simulink model "IM_RFOC_controller_sim"  (R2023a)
settings: Solver=ode23t  StartTime=0.0  StopTime=50  RelTol=1e-3
values from neighbouring files (symbols this model uses):
  B = 0.068    [IM_model_parameters.m]
  f = 50    [IM_model_parameters.m]
  isq_n = 1.278    [IM_model_parameters.m]
  J = 0.4    [IM_model_parameters.m]
  k = 0.009    [IM_model_parameters.m]
  kicdq = 41.5*100    (= 4150)    [IM_model_parameters.m]
  kiw = 0.068*1000    (= 68)    [IM_model_parameters.m]
  kiYr = 17.54286*1000    (= 17542.86)    [IM_model_parameters.m]
  kpcdq = .4425*100    (= 44.25)    [IM_model_parameters.m]
  kpw = 0.4*1000    (= 400)    [IM_model_parameters.m]
  kpYr = 5.71429*1000    (= 5714.29)    [IM_model_parameters.m]
  Lks = Ls- Lm^2/Lr    (= 0.00442538071066)    [IM_model_parameters.m]
  Lm = 57e-3    (= 0.057)    [IM_model_parameters.m]
  np = 3    [IM_model_parameters.m]
  r = 4    [IM_model_parameters.m]
  Rr = 0.175    [IM_model_parameters.m]
  Rs = 0.24    [IM_model_parameters.m]
  vsat = 380    [IM_model_parameters.m]
  Yrd_n = 1.9373    [IM_model_parameters.m]
undefined symbols (not defined in the file or in its folder): j, magnitude
libraries: slpidlib x4, eeTransforms x4, simulink x1
settings Model: Creator=Andrea  LastModifiedBy=Andrea
settings SolverCC: ZeroCrossAlgorithm=Adaptive
settings OptimizationCC: ReuseModelBlockBuffer=off

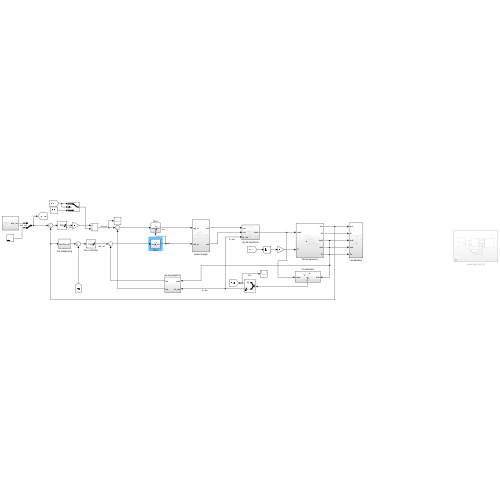
[thumbnail: Simulink's stored preview of the top-level diagram]
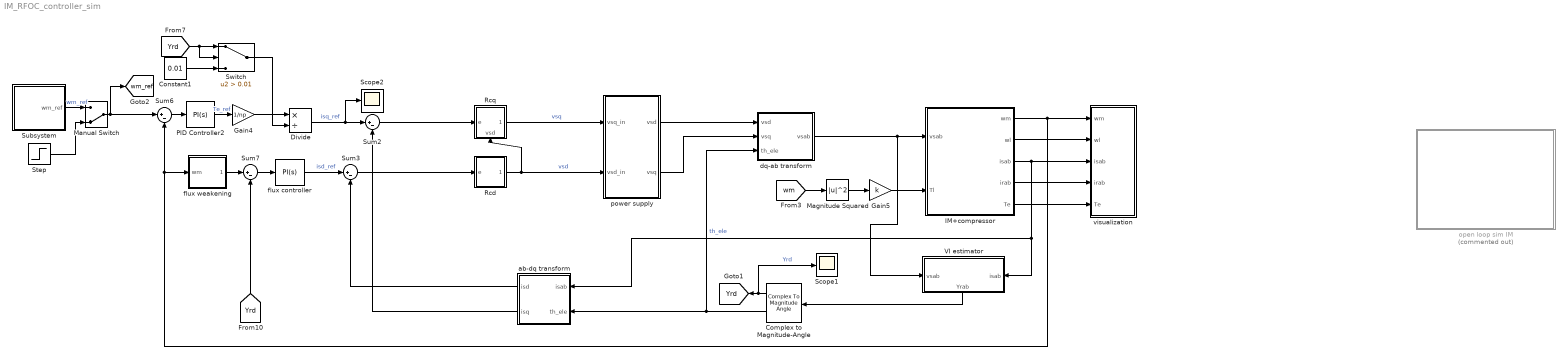
== system IM_RFOC_controller_sim ==
  Complex to Magnitude-Angle : ComplexToMagnitudeAngle
  Constant1 : Constant  Value=0.01
  Divide : Product  Inputs=*/  RndMeth=Zero  SaturateOnIntegerOverflow=on
  Gain4 : Gain  Gain=1/np
  Gain5 : Gain  Gain=k
  IM+compressor : Subsystem
  Magnitude Squared : Math  Operator=magnitude^2
  Manual Switch : ManualSwitch  CurrentSetting=0
  PID Controller2 : slpidlib/PID Controller  Controller=PI  Form=Parallel  TimeDomain=Continuous-time  UseExternalTs=off  SampleTime=-1  IntegratorMethod=Forward Euler  FilterMethod=Forward Euler  ControllerParametersSource=internal  P=kpw  I=kiw  UseKiTs=off  D=0  N=100  UseFilter=on  TunerSelectOption=Transfer Function Based (PID Tuner App)  InitialConditionSource=internal  InitialConditionForIntegrator=0  InitialConditionForFilter=0  DifferentiatorICPrevScaledInput=0  ExternalReset=none  TrackingMode=off  Kt=1  LimitOutput=on  SatLimitsSource=internal  UpperSaturationLimit=1000  LowerSaturationLimit=-1000  LinearizeAsGain=on  AntiWindupMode=back-calculation  Kb=kiw/kpw  LimitIntegrator=off  UpperIntegratorSaturationLimit=inf  LowerIntegratorSaturationLimit=-inf  POutMin=[]  POutMax=[]  IOutMin=[]  IOutMax=[]  DOutMin=[]  DOutMax=[]  NOutMin=[]  NOutMax=[]  SumOutMin=[]  SumOutMax=[]  SaturationOutMin=[]  SaturationOutMax=[]  PParamMin=[]  PParamMax=[]  IParamMin=[]  IParamMax=[]  DParamMin=[]  DParamMax=[]  NParamMin=[]  NParamMax=[]  KbParamMin=[]  KbParamMax=[]  KtParamMin=[]  KtParamMax=[]  KbOutMin=[]  KbOutMax=[]  KtOutMin=[]  KtOutMax=[]  IntegratorOutMin=[]  IntegratorOutMax=[]  FilterOutMin=[]  FilterOutMax=[]  SumI1OutMin=[]  SumI1OutMax=[]  SumI2OutMin=[]  SumI2OutMax=[]  SumI3OutMin=[]  SumI3OutMax=[]  SumI4OutMin=[]  SumI4OutMax=[]  SumDOutMin=[]  SumDOutMax=[]  DifferentiatorOutMin=[]  DifferentiatorOutMax=[]  FilterDiffOutCoefMin=[]  FilterDiffOutCoefMax=[]  ReciprocalOutMin=[]  ReciprocalOutMax=[]  SumDenOutMin=[]  SumDenOutMax=[]  SumNumOutMin=[]  SumNumOutMax=[]  DivideOutMin=[]  DivideOutMax=[]  UdiffTsProdOutMin=[]  UdiffTsProdOutMax=[]  NTsProdOutMin=[]  NTsProdOutMax=[]  UintegralTsProdOutMin=[]  UintegralTsProdOutMax=[]  UngainTsProdOutMin=[]  UngainTsProdOutMax=[]  ClampingZeroOutDataTypeStr=Inherit: Inherit via back propagation  ClampingZeroOutMin=[]  ClampingZeroOutMax=[]  FilterDenConstantOutDataTypeStr=Inherit: Inherit via back propagation  FilterDenConstantOutMin=[]  FilterDenConstantOutMax=[]  PCopyOutDataTypeStr=Inherit: Inherit via back propagation  PCopyOutMin=[]  PCopyOutMax=[]  NCopyOutDataTypeStr=Inherit: Inherit via back propagation  NCopyOutMin=[]  NCopyOutMax=[]  IntegratorContinuousStateAttributes=''  IntegratorStateMustResolveToSignalObject=off  IntegratorRTWStateStorageClass=Auto  FilterContinuousStateAttributes=''  FilterStateMustResolveToSignalObject=off  FilterRTWStateStorageClass=Auto  ParallelPVariant=InternalParameters  IdealPVariant=Disabled  IVariant=InternalParameters  DVariant=Disabled  IntegratorVariant=Continuous  SatVariant=Enabled  AWVariant=BackCalculation  PCopyVariant=Disabled  TRVariant=Disabled  FdbkBlocksVariant=Forward  IdealPFdbkVariant=Disabled  SatFdbkVariant=Disabled  DerivativeFilterVariant=Disabled  NVariant=Disabled  NCopyVariant=Disabled_SignalSpec  FilterICVariant=Disabled  IntegratorICVariant=InternalICs  ExternalResetVariant=Disabled  TRSumVariant=Passthrough  SumFdbkVariant=Disabled  SumVariant=Sum_PI  TsampFilterVariant=InternalTs  TsampNgainVariant=Passthrough  TsampIntegralVariant=Disabled_SignalSpec  ExternalSaturationOutDataTypeStr=Inherit: Same as second input
  Rcd : Subsystem
  Rcq : Subsystem
      settings: PortSchema="{\"entries\":[{\"content\":{\"sides\":[{\"content\":{\"connectorIds\":[\"In1\"]},\"type\":\"ConnectorPlacement.EquallySpacedRectSide\",\"uuid\":\"4a0c1cc3-c5ad-4afb-85ab-da55195444c6\"},{\"content\":{\"connectorIds\":[\"Out1\"],\"side\":\"RIGHT\"},\"type\":\"ConnectorPlacement.EquallySpacedRectSide\",\"uuid\":\"d24be668-1d0c-4d32-ba8c-18ff6b5ffdfe\"},{\"content\":{\"side\":\"TOP\"},\"type\":\"ConnectorPlacement.EquallySpacedRectSide\",\"uuid\":\"149b91f5-2af2-4df5-b968-7fe381dfd022\"},{\"content\":{\"connectorIds\":[\"In2\"],\"side\":\"BOTTOM\"},\"type\":\"ConnectorPlacement.EquallySpacedRectSide\",\"uuid\":\"c725719b-4b0c-406e-92d6-5caa670663a4\"}]},\"type\":\"ConnectorPlacement.EquallySpacedConnector\",\"uuid\":\"0f41f2af-cb74-4ff9-b902-e7fe768cb33d\"}],\"packageUris\":[\"http://schema.mathworks.com/mf0/Connector/R2020b\"],\"version\":\"1.0\"}"
  Scope1 : Scope
  Scope2 : Scope
  Step : Step  Time=2  After=200  SampleTime=0
  Subsystem : Subsystem
  Sum{2..3,6..7} (4 alike) : Sum  Inputs=|+-
  Switch : Switch  Criteria=u2 > Threshold  Threshold=0.01  SaturateOnIntegerOverflow=off  InputSameDT=off
  VI estimator : Subsystem
      settings: PortSchema="{\"entries\":[{\"content\":{\"sides\":[{\"content\":{},\"type\":\"ConnectorPlacement.EquallySpacedRectSide\",\"uuid\":\"e33eea5d-c803-4efd-b963-b28e7fd3b846\"},{\"content\":{\"connectorIds\":[\"Out1\"],\"side\":\"RIGHT\"},\"type\":\"ConnectorPlacement.EquallySpacedRectSide\",\"uuid\":\"16dd9f0c-f93f-4294-bb00-4f02950fe655\"},{\"content\":{\"connectorIds\":[\"In1\"],\"side\":\"TOP\"},\"type\":\"ConnectorPlacement.EquallySpacedRectSide\",\"uuid\":\"0c6e3d24-7610-41dc-8be5-eb5e396d3954\"},{\"content\":{\"connectorIds\":[\"In2\"],\"side\":\"BOTTOM\"},\"type\":\"ConnectorPlacement.EquallySpacedRectSide\",\"uuid\":\"785fd01a-f2d8-4593-9bc3-fce65e17d3d8\"}]},\"type\":\"ConnectorPlacement.EquallySpacedConnector\",\"uuid\":\"dc648cf4-6df6-4217-8a75-6fc5bc573b99\"}],\"packageUris\":[\"http://schema.mathworks.com/mf0/Connector/R2020b\"],\"version\":\"1.0\"}"
  ab-dq transform : Subsystem
  dq-ab transform : Subsystem
  flux controller : slpidlib/PID Controller  Controller=PI  Form=Parallel  TimeDomain=Continuous-time  UseExternalTs=off  SampleTime=-1  IntegratorMethod=Forward Euler  FilterMethod=Forward Euler  ControllerParametersSource=internal  P=kpYr  I=kiYr  UseKiTs=off  D=0  N=100  UseFilter=on  TunerSelectOption=Transfer Function Based (PID Tuner App)  InitialConditionSource=internal  InitialConditionForIntegrator=0  InitialConditionForFilter=0  DifferentiatorICPrevScaledInput=0  ExternalReset=none  TrackingMode=off  Kt=1  LimitOutput=on  SatLimitsSource=internal  UpperSaturationLimit=50  LowerSaturationLimit=-50  LinearizeAsGain=on  AntiWindupMode=back-calculation  Kb=kiYr/kpYr  LimitIntegrator=off  UpperIntegratorSaturationLimit=inf  LowerIntegratorSaturationLimit=-inf  POutMin=[]  POutMax=[]  IOutMin=[]  IOutMax=[]  DOutMin=[]  DOutMax=[]  NOutMin=[]  NOutMax=[]  SumOutMin=[]  SumOutMax=[]  SaturationOutMin=[]  SaturationOutMax=[]  PParamMin=[]  PParamMax=[]  IParamMin=[]  IParamMax=[]  DParamMin=[]  DParamMax=[]  NParamMin=[]  NParamMax=[]  KbParamMin=[]  KbParamMax=[]  KtParamMin=[]  KtParamMax=[]  KbOutMin=[]  KbOutMax=[]  KtOutMin=[]  KtOutMax=[]  IntegratorOutMin=[]  IntegratorOutMax=[]  FilterOutMin=[]  FilterOutMax=[]  SumI1OutMin=[]  SumI1OutMax=[]  SumI2OutMin=[]  SumI2OutMax=[]  SumI3OutMin=[]  SumI3OutMax=[]  SumI4OutMin=[]  SumI4OutMax=[]  SumDOutMin=[]  SumDOutMax=[]  DifferentiatorOutMin=[]  DifferentiatorOutMax=[]  FilterDiffOutCoefMin=[]  FilterDiffOutCoefMax=[]  ReciprocalOutMin=[]  ReciprocalOutMax=[]  SumDenOutMin=[]  SumDenOutMax=[]  SumNumOutMin=[]  SumNumOutMax=[]  DivideOutMin=[]  DivideOutMax=[]  UdiffTsProdOutMin=[]  UdiffTsProdOutMax=[]  NTsProdOutMin=[]  NTsProdOutMax=[]  UintegralTsProdOutMin=[]  UintegralTsProdOutMax=[]  UngainTsProdOutMin=[]  UngainTsProdOutMax=[]  ClampingZeroOutDataTypeStr=Inherit: Inherit via back propagation  ClampingZeroOutMin=[]  ClampingZeroOutMax=[]  FilterDenConstantOutDataTypeStr=Inherit: Inherit via back propagation  FilterDenConstantOutMin=[]  FilterDenConstantOutMax=[]  PCopyOutDataTypeStr=Inherit: Inherit via back propagation  PCopyOutMin=[]  PCopyOutMax=[]  NCopyOutDataTypeStr=Inherit: Inherit via back propagation  NCopyOutMin=[]  NCopyOutMax=[]  IntegratorContinuousStateAttributes=''  IntegratorStateMustResolveToSignalObject=off  IntegratorRTWStateStorageClass=Auto  FilterContinuousStateAttributes=''  FilterStateMustResolveToSignalObject=off  FilterRTWStateStorageClass=Auto  ParallelPVariant=InternalParameters  IdealPVariant=Disabled  IVariant=InternalParameters  DVariant=Disabled  IntegratorVariant=Continuous  SatVariant=Enabled  AWVariant=BackCalculation  PCopyVariant=Disabled  TRVariant=Disabled  FdbkBlocksVariant=Forward  IdealPFdbkVariant=Disabled  SatFdbkVariant=Disabled  DerivativeFilterVariant=Disabled  NVariant=Disabled  NCopyVariant=Disabled_SignalSpec  FilterICVariant=Disabled  IntegratorICVariant=InternalICs  ExternalResetVariant=Disabled  TRSumVariant=Passthrough  SumFdbkVariant=Disabled  SumVariant=Sum_PI  TsampFilterVariant=InternalTs  TsampNgainVariant=Passthrough  TsampIntegralVariant=Disabled_SignalSpec  ExternalSaturationOutDataTypeStr=Inherit: Same as second input
  flux weakening : Subsystem
  open loop sim IM : Subsystem  Commented=on
  power supply : Subsystem
  visualization : Subsystem
  tag scope: Yrd=global, wm_ref=global
  wires:
  VI estimator/1(Yrab) -> Complex to Magnitude-Angle/1
  Complex to Magnitude-Angle/1 -> Scope1/1, [Yrd]  "Yrd"
  Complex to Magnitude-Angle/2 -> dq-ab transform/3(th_ele), ab-dq transform/2(th_ele)  "th_ele"
  flux controller/1 -> Sum3/1  "isd_ref"
  Divide/1 -> Scope2/1, Sum2/1  "isq_ref"
  Gain4/1 -> Divide/1
  PID Controller2/1 -> Gain4/1  "Te_ref"
  Sum7/1 -> flux controller/1
  IM+compressor/3(isab) -> VI estimator/1(isab), ab-dq transform/1(isab), visualization/3(isab)
  [Yrd] -> Switch/2, Switch/1
  Constant1/1 -> Switch/3
  [wm] -> Magnitude Squared/1
  Magnitude Squared/1 -> Gain5/1
  [Yrd] -> Sum7/2
  Sum6/1 -> PID Controller2/1
  IM+compressor/1(wm) -> Sum6/2, flux weakening/1(wm), visualization/1(wm)
  Step/1 -> Manual Switch/2
  Gain5/1 -> IM+compressor/2(Tl)
  flux weakening/1(Yrd_ref) -> Sum7/1
  Manual Switch/1 -> [wm_ref], Sum6/1
  Subsystem/1(wm_ref) -> Manual Switch/1  "wm_ref"
  Sum2/1 -> Rcq/1(e)
  Rcq/1(vsq_ref) -> power supply/1(vsq_in)  "vsq"
  Sum3/1 -> Rcd/1(e)
  dq-ab transform/1(vsab) -> IM+compressor/1(vsab), VI estimator/2(vsab)
  power supply/1(vsd) -> dq-ab transform/1(vsd)
  power supply/2(vsq) -> dq-ab transform/2(vsq)
  ab-dq transform/2(isq) -> Sum2/2
  ab-dq transform/1(isd) -> Sum3/2
  Switch/1 -> Divide/2
  Rcd/1(vsd_ref) -> power supply/2(vsd_in), Rcq/2(vsd)  "vsd"
  IM+compressor/2(wl) -> visualization/2(wl)
  IM+compressor/4(irab) -> visualization/4(irab)
  IM+compressor/5(Te) -> visualization/5(Te)

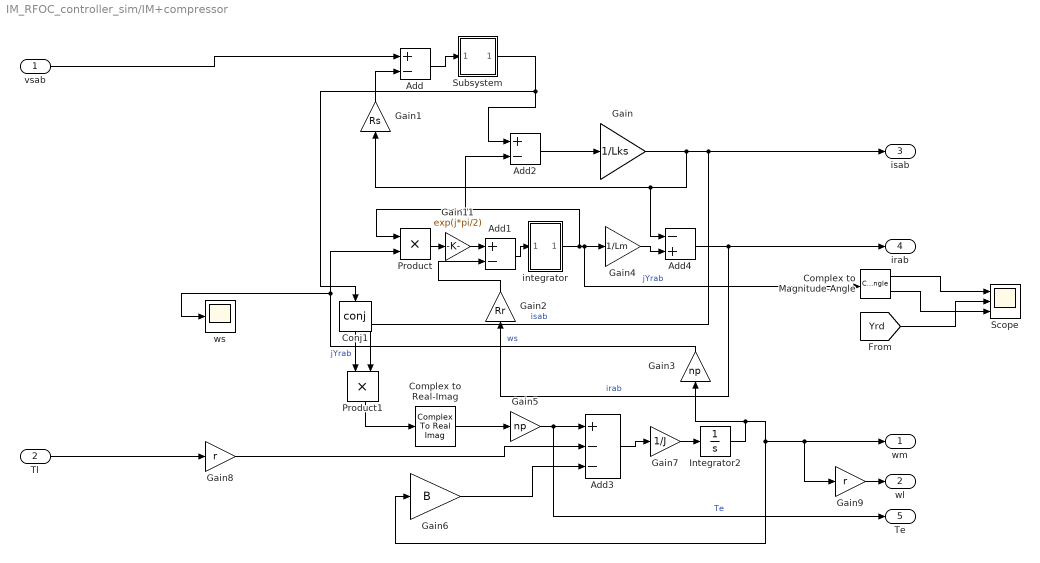
== system IM_RFOC_controller_sim/IM+compressor ==
  vsab : Inport
  Tl : Inport  Port=2
  Add : Sum  Inputs=+-
  Add1 : Sum  Inputs=+-
  Add2 : Sum  Inputs=+-
  Add3 : Sum  Inputs=+--
  Add4 : Sum  Inputs=-+
  Complex to Magnitude-Angle : ComplexToMagnitudeAngle
  Complex to Real-Imag : ComplexToRealImag  Output=Imag
  Conj1 : Math  Operator=conj
  Gain : Gain  Gain=1/Lks
  Gain1 : Gain  Gain=Rs
  Gain11 : Gain  Gain=exp(j*pi/2)
  Gain2 : Gain  Gain=Rr
  Gain3 : Gain  Gain=np
  Gain4 : Gain  Gain=1/Lm
  Gain5 : Gain  Gain=np
  Gain6 : Gain  Gain=B
  Gain7 : Gain  Gain=1/J
  Gain8 : Gain  Gain=r
  Gain9 : Gain  Gain=r
  Integrator2 : Integrator
  Product : Product
  Product1 : Product
  Scope : Scope  NumInputPorts=3
  Subsystem : Subsystem
  integrator : Subsystem
  ws : Scope
  wm : Outport
  wl : Outport  Port=2
  isab : Outport  Port=3
      settings: SignalType=complex
  irab : Outport  Port=4
      settings: SignalType=complex
  Te : Outport  Port=5
  wires:
  Add2/1 -> Gain/1
  Add4/1 -> Gain2/1, irab/1  "irab"
  Gain/1 -> Add4/1, Gain1/1, Product1/2, isab/1  "isab"
  Gain6/1 -> Add3/3
  Gain4/1 -> Add4/2
  integrator/1(Yrab) -> Complex to Magnitude-Angle/1, Gain4/1, Product/1, Add2/2  "jYrab"
  Gain1/1 -> Add/2
  Gain5/1 -> Te/1, Add3/1  "Te"
  Product1/1 -> Complex to Real-Imag/1
  Conj1/1 -> Product1/1  "jYrab"
  Complex to Real-Imag/1 -> Gain5/1
  Gain2/1 -> Add1/2
  Add3/1 -> Gain7/1
  Gain7/1 -> Integrator2/1
  Gain3/1 -> Product/2, ws/1  "ws"
  vsab/1 -> Add/1
  Tl/1 -> Gain8/1
  Add1/1 -> integrator/1(In1)
  Subsystem/1(Ysab) -> Add2/1, Conj1/1
  Add/1 -> Subsystem/1(In1)
  Gain11/1 -> Add1/1
  Product/1 -> Gain11/1
  Gain8/1 -> Add3/2
  Integrator2/1 -> Gain9/1, wm/1, Gain6/1, Gain3/1
  Gain9/1 -> wl/1
  [Yrd] -> Scope/2
  Complex to Magnitude-Angle/1 -> Scope/1
  Complex to Magnitude-Angle/2 -> Scope/3

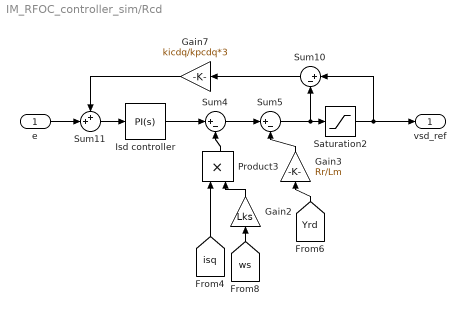
== system IM_RFOC_controller_sim/Rcd ==
  e : Inport
  Gain2 : Gain  Gain=Lks
  Gain3 : Gain  Gain=Rr/Lm
  Gain7 : Gain  Gain=kicdq/kpcdq*3
  Isd controller : slpidlib/PID Controller  Controller=PI  Form=Parallel  TimeDomain=Continuous-time  UseExternalTs=off  SampleTime=-1  IntegratorMethod=Forward Euler  FilterMethod=Forward Euler  ControllerParametersSource=internal  P=kpcdq  I=kicdq  UseKiTs=off  D=0  N=100  UseFilter=on  TunerSelectOption=Transfer Function Based (PID Tuner App)  InitialConditionSource=internal  InitialConditionForIntegrator=0  InitialConditionForFilter=0  DifferentiatorICPrevScaledInput=0  ExternalReset=none  TrackingMode=off  Kt=1  LimitOutput=off  SatLimitsSource=internal  UpperSaturationLimit=vsat*sqrt(3)/sqrt(2)  LowerSaturationLimit=-vsat*sqrt(3)/sqrt(2)  LinearizeAsGain=on  AntiWindupMode=back-calculation  Kb=kicdq/kpcdq  LimitIntegrator=off  UpperIntegratorSaturationLimit=inf  LowerIntegratorSaturationLimit=-inf  POutMin=[]  POutMax=[]  IOutMin=[]  IOutMax=[]  DOutMin=[]  DOutMax=[]  NOutMin=[]  NOutMax=[]  SumOutMin=[]  SumOutMax=[]  SaturationOutMin=[]  SaturationOutMax=[]  PParamMin=[]  PParamMax=[]  IParamMin=[]  IParamMax=[]  DParamMin=[]  DParamMax=[]  NParamMin=[]  NParamMax=[]  KbParamMin=[]  KbParamMax=[]  KtParamMin=[]  KtParamMax=[]  KbOutMin=[]  KbOutMax=[]  KtOutMin=[]  KtOutMax=[]  IntegratorOutMin=[]  IntegratorOutMax=[]  FilterOutMin=[]  FilterOutMax=[]  SumI1OutMin=[]  SumI1OutMax=[]  SumI2OutMin=[]  SumI2OutMax=[]  SumI3OutMin=[]  SumI3OutMax=[]  SumI4OutMin=[]  SumI4OutMax=[]  SumDOutMin=[]  SumDOutMax=[]  DifferentiatorOutMin=[]  DifferentiatorOutMax=[]  FilterDiffOutCoefMin=[]  FilterDiffOutCoefMax=[]  ReciprocalOutMin=[]  ReciprocalOutMax=[]  SumDenOutMin=[]  SumDenOutMax=[]  SumNumOutMin=[]  SumNumOutMax=[]  DivideOutMin=[]  DivideOutMax=[]  UdiffTsProdOutMin=[]  UdiffTsProdOutMax=[]  NTsProdOutMin=[]  NTsProdOutMax=[]  UintegralTsProdOutMin=[]  UintegralTsProdOutMax=[]  UngainTsProdOutMin=[]  UngainTsProdOutMax=[]  ClampingZeroOutDataTypeStr=Inherit: Inherit via back propagation  ClampingZeroOutMin=[]  ClampingZeroOutMax=[]  FilterDenConstantOutDataTypeStr=Inherit: Inherit via back propagation  FilterDenConstantOutMin=[]  FilterDenConstantOutMax=[]  PCopyOutDataTypeStr=Inherit: Inherit via back propagation  PCopyOutMin=[]  PCopyOutMax=[]  NCopyOutDataTypeStr=Inherit: Inherit via back propagation  NCopyOutMin=[]  NCopyOutMax=[]  IntegratorContinuousStateAttributes=''  IntegratorStateMustResolveToSignalObject=off  IntegratorRTWStateStorageClass=Auto  FilterContinuousStateAttributes=''  FilterStateMustResolveToSignalObject=off  FilterRTWStateStorageClass=Auto  ParallelPVariant=InternalParameters  IdealPVariant=Disabled  IVariant=InternalParameters  DVariant=Disabled  IntegratorVariant=Continuous  SatVariant=Disabled  AWVariant=Passthrough  PCopyVariant=Disabled  TRVariant=Disabled  FdbkBlocksVariant=Forward  IdealPFdbkVariant=Disabled  SatFdbkVariant=Disabled  DerivativeFilterVariant=Disabled  NVariant=Disabled  NCopyVariant=Disabled_SignalSpec  FilterICVariant=Disabled  IntegratorICVariant=InternalICs  ExternalResetVariant=Disabled  TRSumVariant=Passthrough  SumFdbkVariant=Disabled  SumVariant=Sum_PI  TsampFilterVariant=InternalTs  TsampNgainVariant=Passthrough  TsampIntegralVariant=Disabled_SignalSpec  ExternalSaturationOutDataTypeStr=Inherit: Same as second input
  Product3 : Product
  Saturation2 : Saturate  UpperLimit=vsat*sqrt(3)/sqrt(2)  LowerLimit=-vsat*sqrt(3)/sqrt(2)
  Sum10 : Sum  Inputs=|+-
  Sum11 : Sum  Inputs=++|
  Sum4 : Sum  Inputs=|+-
  Sum5 : Sum  Inputs=|+-
  vsd_ref : Outport
  wires:
  Gain7/1 -> Sum11/1
  Saturation2/1 -> vsd_ref/1, Sum10/1
  [isq] -> Product3/1
  Isd controller/1 -> Sum4/1
  Sum11/1 -> Isd controller/1
  Sum4/1 -> Sum5/1
  e/1 -> Sum11/2
  Sum5/1 -> Saturation2/1, Sum10/2
  Gain2/1 -> Product3/2
  Sum10/1 -> Gain7/1
  Product3/1 -> Sum4/2
  [ws] -> Gain2/1
  Gain3/1 -> Sum5/2
  [Yrd] -> Gain3/1

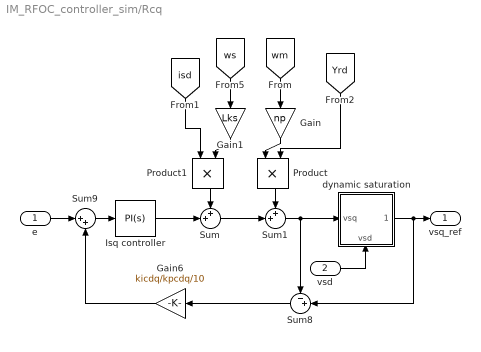
== system IM_RFOC_controller_sim/Rcq ==
  e : Inport
  vsd : Inport  Port=2
  Gain : Gain  Gain=np
  Gain1 : Gain  Gain=Lks
  Gain6 : Gain  Gain=kicdq/kpcdq/10
  Isq controller : slpidlib/PID Controller  Controller=PI  Form=Parallel  TimeDomain=Continuous-time  UseExternalTs=off  SampleTime=-1  IntegratorMethod=Forward Euler  FilterMethod=Forward Euler  ControllerParametersSource=internal  P=kpcdq  I=kicdq  UseKiTs=off  D=0  N=100  UseFilter=on  TunerSelectOption=Transfer Function Based (PID Tuner App)  InitialConditionSource=internal  InitialConditionForIntegrator=0  InitialConditionForFilter=0  DifferentiatorICPrevScaledInput=0  ExternalReset=none  TrackingMode=off  Kt=1  LimitOutput=off  SatLimitsSource=internal  UpperSaturationLimit=vsat*sqrt(3)/sqrt(2)  LowerSaturationLimit=-vsat*sqrt(3)/sqrt(2)  LinearizeAsGain=on  AntiWindupMode=back-calculation  Kb=kicdq/kpcdq  LimitIntegrator=off  UpperIntegratorSaturationLimit=inf  LowerIntegratorSaturationLimit=-inf  POutMin=[]  POutMax=[]  IOutMin=[]  IOutMax=[]  DOutMin=[]  DOutMax=[]  NOutMin=[]  NOutMax=[]  SumOutMin=[]  SumOutMax=[]  SaturationOutMin=[]  SaturationOutMax=[]  PParamMin=[]  PParamMax=[]  IParamMin=[]  IParamMax=[]  DParamMin=[]  DParamMax=[]  NParamMin=[]  NParamMax=[]  KbParamMin=[]  KbParamMax=[]  KtParamMin=[]  KtParamMax=[]  KbOutMin=[]  KbOutMax=[]  KtOutMin=[]  KtOutMax=[]  IntegratorOutMin=[]  IntegratorOutMax=[]  FilterOutMin=[]  FilterOutMax=[]  SumI1OutMin=[]  SumI1OutMax=[]  SumI2OutMin=[]  SumI2OutMax=[]  SumI3OutMin=[]  SumI3OutMax=[]  SumI4OutMin=[]  SumI4OutMax=[]  SumDOutMin=[]  SumDOutMax=[]  DifferentiatorOutMin=[]  DifferentiatorOutMax=[]  FilterDiffOutCoefMin=[]  FilterDiffOutCoefMax=[]  ReciprocalOutMin=[]  ReciprocalOutMax=[]  SumDenOutMin=[]  SumDenOutMax=[]  SumNumOutMin=[]  SumNumOutMax=[]  DivideOutMin=[]  DivideOutMax=[]  UdiffTsProdOutMin=[]  UdiffTsProdOutMax=[]  NTsProdOutMin=[]  NTsProdOutMax=[]  UintegralTsProdOutMin=[]  UintegralTsProdOutMax=[]  UngainTsProdOutMin=[]  UngainTsProdOutMax=[]  ClampingZeroOutDataTypeStr=Inherit: Inherit via back propagation  ClampingZeroOutMin=[]  ClampingZeroOutMax=[]  FilterDenConstantOutDataTypeStr=Inherit: Inherit via back propagation  FilterDenConstantOutMin=[]  FilterDenConstantOutMax=[]  PCopyOutDataTypeStr=Inherit: Inherit via back propagation  PCopyOutMin=[]  PCopyOutMax=[]  NCopyOutDataTypeStr=Inherit: Inherit via back propagation  NCopyOutMin=[]  NCopyOutMax=[]  IntegratorContinuousStateAttributes=''  IntegratorStateMustResolveToSignalObject=off  IntegratorRTWStateStorageClass=Auto  FilterContinuousStateAttributes=''  FilterStateMustResolveToSignalObject=off  FilterRTWStateStorageClass=Auto  ParallelPVariant=InternalParameters  IdealPVariant=Disabled  IVariant=InternalParameters  DVariant=Disabled  IntegratorVariant=Continuous  SatVariant=Disabled  AWVariant=Passthrough  PCopyVariant=Disabled  TRVariant=Disabled  FdbkBlocksVariant=Forward  IdealPFdbkVariant=Disabled  SatFdbkVariant=Disabled  DerivativeFilterVariant=Disabled  NVariant=Disabled  NCopyVariant=Disabled_SignalSpec  FilterICVariant=Disabled  IntegratorICVariant=InternalICs  ExternalResetVariant=Disabled  TRSumVariant=Passthrough  SumFdbkVariant=Disabled  SumVariant=Sum_PI  TsampFilterVariant=InternalTs  TsampNgainVariant=Passthrough  TsampIntegralVariant=Disabled_SignalSpec  ExternalSaturationOutDataTypeStr=Inherit: Same as second input
  Product : Product
  Product1 : Product
  Sum : Sum  Inputs=++|
  Sum1 : Sum  Inputs=++|
  Sum8 : Sum  Inputs=-+|
  Sum9 : Sum  Inputs=|++
  dynamic saturation : Subsystem
      settings: PortSchema="{\"entries\":[{\"content\":{\"sides\":[{\"content\":{\"connectorIds\":[\"In1\"]},\"type\":\"ConnectorPlacement.EquallySpacedRectSide\",\"uuid\":\"702056da-27ae-4f36-9152-163964513796\"},{\"content\":{\"connectorIds\":[\"Out1\"],\"side\":\"RIGHT\"},\"type\":\"ConnectorPlacement.EquallySpacedRectSide\",\"uuid\":\"238bf341-9bee-4b7b-8f4c-7a05bcb8c6b9\"},{\"content\":{\"side\":\"TOP\"},\"type\":\"ConnectorPlacement.EquallySpacedRectSide\",\"uuid\":\"862e1a3e-9d35-426a-9047-2748dbaff7d6\"},{\"content\":{\"connectorIds\":[\"In2\"],\"side\":\"BOTTOM\"},\"type\":\"ConnectorPlacement.EquallySpacedRectSide\",\"uuid\":\"64e0a315-4bd3-4c8c-8d98-cee2641e021c\"}]},\"type\":\"ConnectorPlacement.EquallySpacedConnector\",\"uuid\":\"9e7181e3-db27-40e9-92e7-7d0bed89505e\"}],\"packageUris\":[\"http://schema.mathworks.com/mf0/Connector/R2020b\"],\"version\":\"1.0\"}"
  vsq_ref : Outport
  wires:
  dynamic saturation/1(vsq_ref) -> Sum8/2, vsq_ref/1
  [Yrd] -> Product/2
  Product1/1 -> Sum/1
  [ws] -> Gain1/1
  Sum9/1 -> Isq controller/1
  vsd/1 -> dynamic saturation/2(vsd)
  Gain6/1 -> Sum9/2
  Sum/1 -> Sum1/2
  Isq controller/1 -> Sum/2
  Sum8/1 -> Gain6/1
  [wm] -> Gain/1
  Gain/1 -> Product/1
  Gain1/1 -> Product1/2
  Product/1 -> Sum1/1
  [isd] -> Product1/1
  Sum1/1 -> Sum8/1, dynamic saturation/1(vsq)
  e/1 -> Sum9/1

== system IM_RFOC_controller_sim/Subsystem ==
  Clock : Clock
  MATLAB Function : MATLAB Function  TreatAsAtomicUnit=on
  Scope : Scope
  Sum : Sum  Inputs=|+-
  Ta Yr : Constant  Value=0.04
  wm_ref : Outport
  wires:
  Clock/1 -> Sum/1
  MATLAB Function/1(y) -> Scope/1, wm_ref/1
  Ta Yr/1 -> Sum/2
  Sum/1 -> MATLAB Function/1(t)

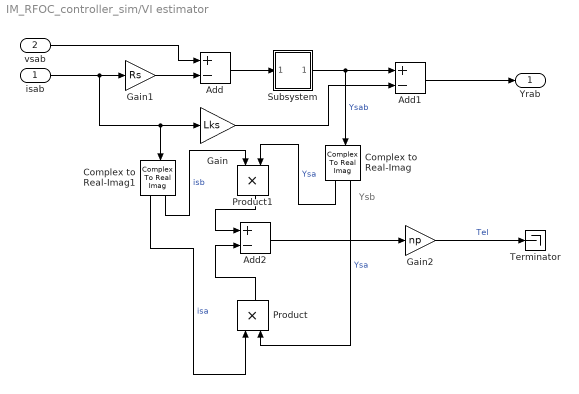
== system IM_RFOC_controller_sim/VI estimator ==
  note: Ysb
  isab : Inport
  vsab : Inport  Port=2
  Add : Sum  Inputs=+-
  Add1 : Sum  Inputs=+-
  Add2 : Sum  Inputs=+-
  Complex to Real-Imag : ComplexToRealImag
  Complex to Real-Imag1 : ComplexToRealImag
  Gain : Gain  Gain=Lks
  Gain1 : Gain  Gain=Rs
  Gain2 : Gain  Gain=np
  Product : Product
  Product1 : Product
  Subsystem : Subsystem
  Terminator : Terminator
  Yrab : Outport
  wires:
  Subsystem/1(Ysab) -> Complex to Real-Imag/1, Add1/1  "Ysab"
  Add/1 -> Subsystem/1(In1)
  Add1/1 -> Yrab/1
  vsab/1 -> Add/1
  Gain1/1 -> Add/2
  Gain/1 -> Add1/2
  isab/1 -> Complex to Real-Imag1/1, Gain/1, Gain1/1
  Complex to Real-Imag/1 -> Product1/2  "Ysa"
  Complex to Real-Imag/2 -> Product/2  "Ysa"
  Complex to Real-Imag1/1 -> Product/1  "isa"
  Product1/1 -> Add2/1
  Product/1 -> Add2/2
  Add2/1 -> Gain2/1
  Gain2/1 -> Terminator/1  "Tel"
  Complex to Real-Imag1/2 -> Product1/1  "isb"

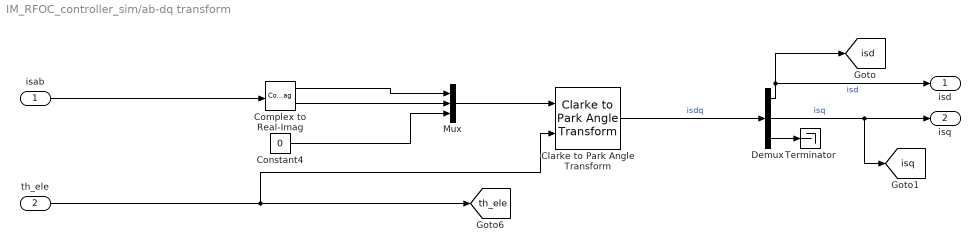
== system IM_RFOC_controller_sim/ab-dq transform ==
  isab : Inport
  th_ele : Inport  Port=2
  Clarke to Park Angle Transform : eeTransforms/Clarke to Park Angle Transform  AxisAlignment=D-axis
      settings: LibrarySourceBlock=|
      | ee_sl_lib/Mathematical
      | Transforms/Clarke to Park
      | Angle Transform
  Complex to Real-Imag : ComplexToRealImag
  Constant4 : Constant  Value=0
  Demux : Demux  Outputs=3
  Mux : Mux  Inputs=3
  Terminator : Terminator
  isd : Outport
  isq : Outport  Port=2
  tag scope: isd=global, isq=global, th_ele=global
  wires:
  th_ele/1 -> Clarke to Park Angle Transform/2, [th_ele]
  Demux/1 -> [isd], isd/1  "isd"
  Demux/3 -> Terminator/1
  Complex to Real-Imag/1 -> Mux/1
  Constant4/1 -> Mux/3
  Complex to Real-Imag/2 -> Mux/2
  Clarke to Park Angle Transform/1 -> Demux/1  "isdq"
  Mux/1 -> Clarke to Park Angle Transform/1
  Demux/2 -> [isq], isq/1  "isq"
  isab/1 -> Complex to Real-Imag/1

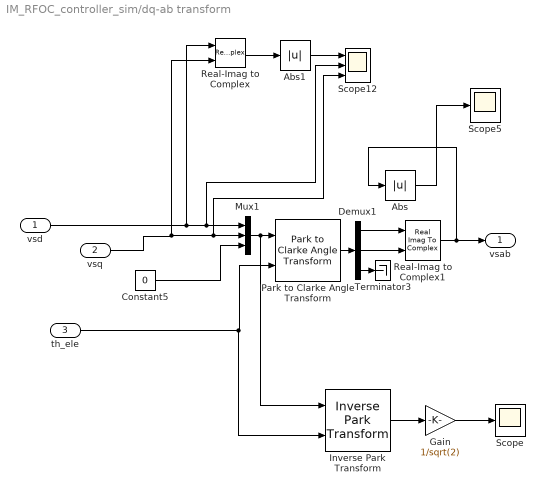
== system IM_RFOC_controller_sim/dq-ab transform ==
  vsd : Inport
  vsq : Inport  Port=2
  th_ele : Inport  Port=3
  Abs : Abs  SaturateOnIntegerOverflow=off
  Abs1 : Abs  SaturateOnIntegerOverflow=off
  Constant5 : Constant  Value=0
  Demux1 : Demux  Outputs=3
  Gain : Gain  Gain=1/sqrt(2)
  Inverse Park Transform : eeTransforms/Inverse Park Transform  AxisAlignment=D-axis  PowerInvariant=on
      settings: LibrarySourceBlock=|
      | ee_sl_lib/Mathematical
      | Transforms/Inverse
      | Park Transform
  Mux1 : Mux  Inputs=3
  Park to Clarke Angle Transform : eeTransforms/Park to Clarke Angle Transform  AxisAlignment=D-axis
      settings: LibrarySourceBlock=|
      | ee_sl_lib/Mathematical
      | Transforms/Park to Clarke
      | Angle Transform
  Real-Imag to Complex : RealImagToComplex
  Real-Imag to Complex1 : RealImagToComplex
  Scope : Scope
  Scope12 : Scope  NumInputPorts=3
  Scope5 : Scope
  Terminator3 : Terminator
  vsab : Outport
  wires:
  Park to Clarke Angle Transform/1 -> Demux1/1
  vsd/1 -> Real-Imag to Complex/1, Scope12/2, Mux1/1
  vsq/1 -> Scope12/3, Mux1/2, Real-Imag to Complex/2
  Demux1/3 -> Terminator3/1
  Constant5/1 -> Mux1/3
  Real-Imag to Complex1/1 -> vsab/1, Abs/1
  Abs1/1 -> Scope12/1
  Demux1/1 -> Real-Imag to Complex1/1
  Real-Imag to Complex/1 -> Abs1/1
  Abs/1 -> Scope5/1
  Demux1/2 -> Real-Imag to Complex1/2
  Mux1/1 -> Inverse Park Transform/1, Park to Clarke Angle Transform/1
  th_ele/1 -> Inverse Park Transform/2, Park to Clarke Angle Transform/2
  Inverse Park Transform/1 -> Gain/1
  Gain/1 -> Scope/1

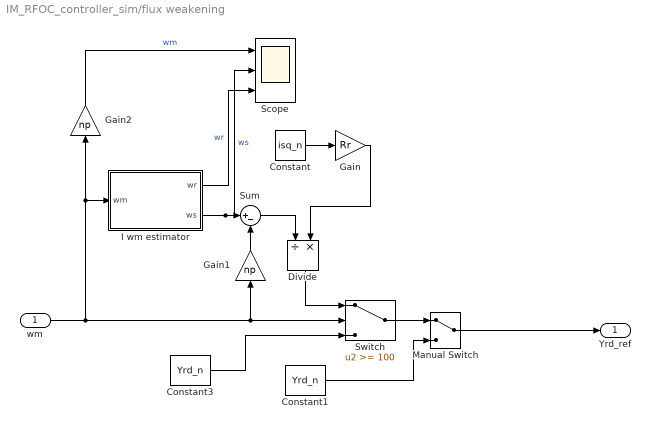
== system IM_RFOC_controller_sim/flux weakening ==
  wm : Inport
  Constant : Constant  Value=isq_n
  Constant1 : Constant  Value=Yrd_n
  Constant3 : Constant  Value=Yrd_n
  Divide : Product  Inputs=/*
  Gain : Gain  Gain=Rr
  Gain1 : Gain  Gain=np
  Gain2 : Gain  Gain=np
  I wm estimator : Subsystem
  Manual Switch : ManualSwitch
  Scope : Scope  NumInputPorts=3
  Sum : Sum  Inputs=|+-
  Switch : Switch  Threshold=100  SaturateOnIntegerOverflow=off  InputSameDT=off
  Yrd_ref : Outport
  wires:
  Constant3/1 -> Switch/3
  Sum/1 -> Divide/1
  Divide/1 -> Switch/1
  Constant/1 -> Gain/1
  Gain/1 -> Divide/2
  Gain1/1 -> Sum/2
  Switch/1 -> Manual Switch/1
  Constant1/1 -> Manual Switch/2
  I wm estimator/2(ws) -> Scope/2, Sum/1  "ws"
  wm/1 -> Gain2/1, I wm estimator/1(wm), Gain1/1, Switch/2
  Manual Switch/1 -> Yrd_ref/1
  I wm estimator/1(wr) -> Scope/3  "wr"
  Gain2/1 -> Scope/1  "wm"

== system IM_RFOC_controller_sim/open loop sim IM ==
  Constant4 : Constant  Value=0
  IM : Subsystem
  Supplying at Vn : Subsystem
  VI estimator4 : Subsystem
      settings: PortSchema="{\"entries\":[{\"content\":{\"sides\":[{\"content\":{},\"type\":\"ConnectorPlacement.EquallySpacedRectSide\",\"uuid\":\"e33eea5d-c803-4efd-b963-b28e7fd3b846\"},{\"content\":{\"connectorIds\":[\"Out1\",\"Out2\",\"Out3\"],\"side\":\"RIGHT\"},\"type\":\"ConnectorPlacement.EquallySpacedRectSide\",\"uuid\":\"16dd9f0c-f93f-4294-bb00-4f02950fe655\"},{\"content\":{\"connectorIds\":[\"In1\"],\"side\":\"TOP\"},\"type\":\"ConnectorPlacement.EquallySpacedRectSide\",\"uuid\":\"0c6e3d24-7610-41dc-8be5-eb5e396d3954\"},{\"content\":{\"connectorIds\":[\"In2\"],\"side\":\"BOTTOM\"},\"type\":\"ConnectorPlacement.EquallySpacedRectSide\",\"uuid\":\"785fd01a-f2d8-4593-9bc3-fce65e17d3d8\"}]},\"type\":\"ConnectorPlacement.EquallySpacedConnector\",\"uuid\":\"dc648cf4-6df6-4217-8a75-6fc5bc573b99\"}],\"packageUris\":[\"http://schema.mathworks.com/mf0/Connector/R2020b\"],\"version\":\"1.0\"}"
  Visualization : Subsystem
  wires:
  IM/2(isab) -> VI estimator4/1(isab), Visualization/2(isab)
  Constant4/1 -> IM/2(Tl)
  Supplying at Vn/1(AlphaBeta0) -> VI estimator4/2(vsab), IM/1(vsab)
  IM/1(wm) -> Visualization/1(wm)
  IM/3(irab) -> Visualization/3(irab)
  IM/4(Te) -> Visualization/4(Te)
  VI estimator4/3(Ysab) -> Visualization/5(Ysab)
  VI estimator4/2(Yrab) -> Visualization/6(Yrab)

== system IM_RFOC_controller_sim/power supply ==
  vsq_in : Inport
  vsd_in : Inport  Port=2
  Scope : Scope  NumInputPorts=2
  vsd : Outport
  vsq : Outport  Port=2
  wires:
  vsq_in/1 -> Scope/1, vsq/1
  vsd_in/1 -> Scope/2, vsd/1

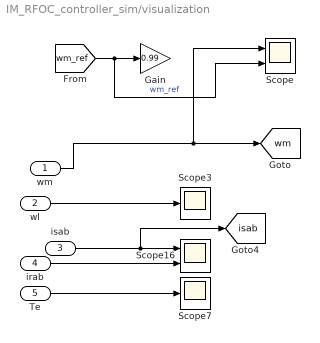
== system IM_RFOC_controller_sim/visualization ==
  wm : Inport
  wl : Inport  Port=2
  isab : Inport  Port=3
  irab : Inport  Port=4
  Te : Inport  Port=5
  Gain : Gain  Gain=0.99
  Scope : Scope  NumInputPorts=2
  Scope16 : Scope  NumInputPorts=2
  Scope3 : Scope
  Scope7 : Scope
  tag scope: isab=global, wm=global
  wires:
  irab/1 -> Scope16/2
  Te/1 -> Scope7/1
  wm/1 -> [wm], Scope/1
  wl/1 -> Scope3/1
  isab/1 -> [isab], Scope16/1
  [wm_ref] -> Scope/2, Gain/1  "wm_ref"

== system IM_RFOC_controller_sim/IM+compressor/Subsystem ==
  note: to avoid numerical issues
  In1 : Inport
  Complex to Real-Imag6 : ComplexToRealImag
  Integrator3 : Integrator
  Integrator4 : Integrator
  Real-Imag to Complex : RealImagToComplex
  Ysab : Outport
  wires:
  In1/1 -> Complex to Real-Imag6/1
  Complex to Real-Imag6/2 -> Integrator4/1
  Complex to Real-Imag6/1 -> Integrator3/1
  Integrator3/1 -> Real-Imag to Complex/1
  Real-Imag to Complex/1 -> Ysab/1  "Ysab"
  Integrator4/1 -> Real-Imag to Complex/2

== system IM_RFOC_controller_sim/IM+compressor/integrator ==
  In1 : Inport
  Complex to Real-Imag7 : ComplexToRealImag
  Integrator1 : Integrator
  Integrator5 : Integrator
  Real-Imag to Complex1 : RealImagToComplex
  Yrab : Outport
  wires:
  Complex to Real-Imag7/2 -> Integrator5/1
  Integrator1/1 -> Real-Imag to Complex1/1
  Real-Imag to Complex1/1 -> Yrab/1  "Yrab"
  Integrator5/1 -> Real-Imag to Complex1/2
  Complex to Real-Imag7/1 -> Integrator1/1
  In1/1 -> Complex to Real-Imag7/1

== system IM_RFOC_controller_sim/Rcq/dynamic saturation ==
  vsq : Inport
  vsd : Inport  Port=2
  Constant : Constant  Value=vsat^2*3/2*2
  Gain : Gain  Gain=-1
  Magnitude Squared : Math  Operator=magnitude^2
  Saturation : Saturate  UpperLimit=650  LowerLimit=-650
  Saturation Dynamic : simulink/Discontinuities/Saturation Dynamic  OutMin=[]  OutMax=[]  OutDataTypeStr=Inherit: Same as second input  OutDataType=fixdt(1, 16)  OutScaling=2^-10  DoSatur=off
  Scope : Scope  NumInputPorts=2
  Square Root : Sqrt
  Sum12 : Sum  Inputs=|+-
  vsq_ref : Outport
  wires:
  Constant/1 -> Sum12/1
  Saturation Dynamic/1 -> vsq_ref/1
  vsd/1 -> Magnitude Squared/1
  Magnitude Squared/1 -> Sum12/2
  Sum12/1 -> Square Root/1
  Square Root/1 -> Scope/1, Gain/1, Saturation Dynamic/1
  Gain/1 -> Scope/2, Saturation Dynamic/3
  vsq/1 -> Saturation/1
  Saturation/1 -> Saturation Dynamic/2

== system IM_RFOC_controller_sim/VI estimator/Subsystem ==
  note: to avoid numerical issues
  In1 : Inport
  Complex to Real-Imag6 : ComplexToRealImag
  Integrator3 : Integrator
  Integrator4 : Integrator
  Real-Imag to Complex : RealImagToComplex
  Ysab : Outport
  wires:
  In1/1 -> Complex to Real-Imag6/1
  Complex to Real-Imag6/2 -> Integrator4/1
  Complex to Real-Imag6/1 -> Integrator3/1
  Integrator3/1 -> Real-Imag to Complex/1
  Real-Imag to Complex/1 -> Ysab/1  "Ysab"
  Integrator4/1 -> Real-Imag to Complex/2

== system IM_RFOC_controller_sim/flux weakening/I wm estimator ==
  wm : Inport
  Add : Sum
  Constant : Constant  Value=0.00001
  Divide : Product  Inputs=/*
  Gain : Gain  Gain=Rr
  Gain1 : Gain  Gain=np
  Sum : Sum  Inputs=|++
  Transfer Fcn : TransferFcn  Numerator=[Rr]  Denominator=[1 Rr/Lm]
  wr : Outport
  ws : Outport  Port=2
  tag scope: ws=global
  wires:
  Gain1/1 -> Add/2
  wm/1 -> Gain1/1
  Gain/1 -> Divide/2
  Add/1 -> [ws], ws/1
  Divide/1 -> wr/1, Add/1
  Constant/1 -> Sum/2
  Sum/1 -> Divide/1
  [isd] -> Transfer Fcn/1
  [isq] -> Gain/1
  Transfer Fcn/1 -> Sum/1

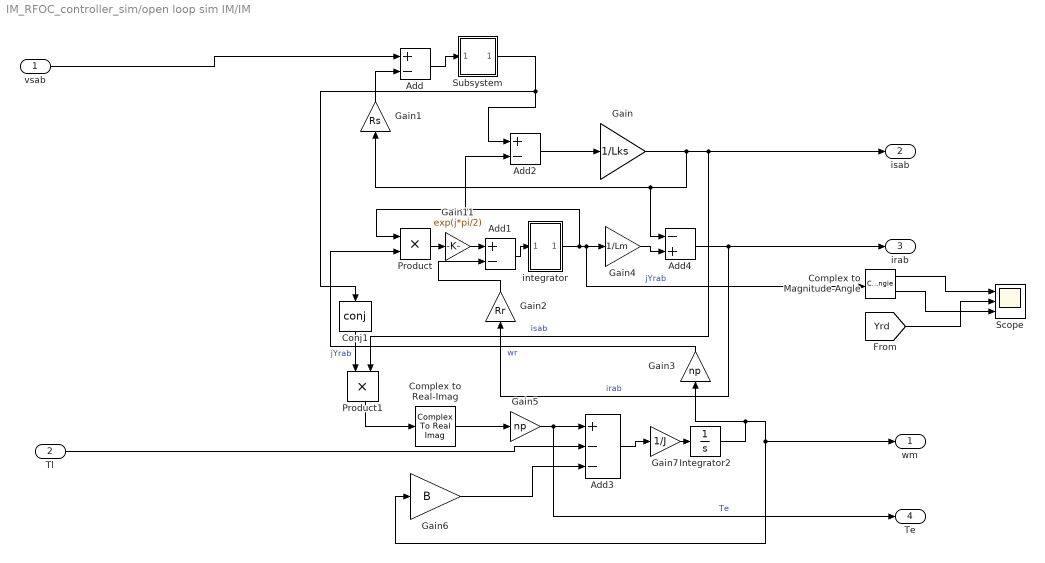
== system IM_RFOC_controller_sim/open loop sim IM/IM ==
  vsab : Inport
  Tl : Inport  Port=2
  Add : Sum  Inputs=+-
  Add1 : Sum  Inputs=+-
  Add2 : Sum  Inputs=+-
  Add3 : Sum  Inputs=+--
  Add4 : Sum  Inputs=-+
  Complex to Magnitude-Angle : ComplexToMagnitudeAngle
  Complex to Real-Imag : ComplexToRealImag  Output=Imag
  Conj1 : Math  Operator=conj
  Gain : Gain  Gain=1/Lks
  Gain1 : Gain  Gain=Rs
  Gain11 : Gain  Gain=exp(j*pi/2)
  Gain2 : Gain  Gain=Rr
  Gain3 : Gain  Gain=np
  Gain4 : Gain  Gain=1/Lm
  Gain5 : Gain  Gain=np
  Gain6 : Gain  Gain=B
  Gain7 : Gain  Gain=1/J
  Integrator2 : Integrator
  Product : Product
  Product1 : Product
  Scope : Scope  NumInputPorts=3
  Subsystem : Subsystem
  integrator : Subsystem
  wm : Outport
  isab : Outport  Port=2
      settings: SignalType=complex
  irab : Outport  Port=3
      settings: SignalType=complex
  Te : Outport  Port=4
  wires:
  Add2/1 -> Gain/1
  Add4/1 -> Gain2/1, irab/1  "irab"
  Gain/1 -> Add4/1, Gain1/1, Product1/2, isab/1  "isab"
  Gain6/1 -> Add3/3
  Gain4/1 -> Add4/2
  Gain1/1 -> Add/2
  Gain5/1 -> Add3/1, Te/1  "Te"
  Product1/1 -> Complex to Real-Imag/1
  Conj1/1 -> Product1/1  "jYrab"
  Complex to Real-Imag/1 -> Gain5/1
  Gain2/1 -> Add1/2
  Add3/1 -> Gain7/1
  Gain7/1 -> Integrator2/1
  Gain3/1 -> Product/2  "wr"
  vsab/1 -> Add/1
  Tl/1 -> Add3/2
  Integrator2/1 -> wm/1, Gain6/1, Gain3/1
  Add1/1 -> integrator/1(In1)
  Add/1 -> Subsystem/1(In1)
  Gain11/1 -> Add1/1
  Product/1 -> Gain11/1
  Complex to Magnitude-Angle/2 -> Scope/3
  [Yrd] -> Scope/2
  integrator/1(Yrab) -> Product/1, Add2/2, Complex to Magnitude-Angle/1, Gain4/1  "jYrab"
  Complex to Magnitude-Angle/1 -> Scope/1
  Subsystem/1(Ysab) -> Add2/1, Conj1/1

== system IM_RFOC_controller_sim/open loop sim IM/Supplying at Vn ==
  note: phasor
  note: ab0 ref sys
  Clarke Transform : eeTransforms/Clarke Transform  PowerInvariant=on
      settings: LibrarySourceBlock=|
      | ee_sl_lib/Mathematical
      | Transforms/Clarke Transform
  Demux : Demux  Outputs=3
  Mux : Mux  Inputs=3
  Real-Imag to Complex : RealImagToComplex
  Sine Wave : Sin  Amplitude=380*sqrt(2)  Frequency=f*2*pi  SampleTime=0
  Sine Wave1 : Sin  Amplitude=380*sqrt(2)  Frequency=f*2*pi  Phase=-2/3*pi  SampleTime=0
  Sine Wave2 : Sin  Amplitude=380*sqrt(2)  Frequency=f*2*pi  Phase=-4/3*pi  SampleTime=0
  AlphaBeta0 : Outport
  wires:
  Sine Wave/1 -> Mux/1
  Mux/1 -> Clarke Transform/1
  Sine Wave2/1 -> Mux/3
  Sine Wave1/1 -> Mux/2
  Demux/2 -> Real-Imag to Complex/2
  Clarke Transform/1 -> Demux/1
  Demux/1 -> Real-Imag to Complex/1
  Real-Imag to Complex/1 -> AlphaBeta0/1

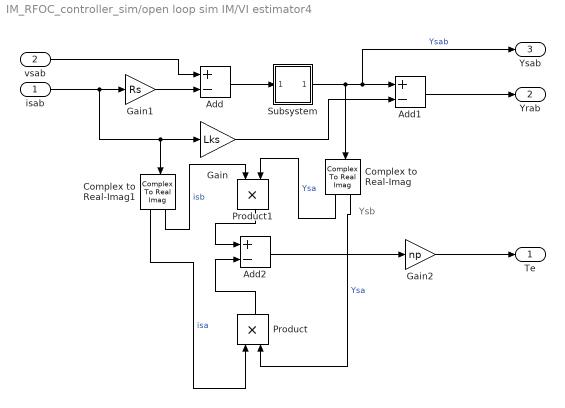
== system IM_RFOC_controller_sim/open loop sim IM/VI estimator4 ==
  note: Ysb
  isab : Inport
  vsab : Inport  Port=2
  Add : Sum  Inputs=+-
  Add1 : Sum  Inputs=+-
  Add2 : Sum  Inputs=+-
  Complex to Real-Imag : ComplexToRealImag
  Complex to Real-Imag1 : ComplexToRealImag
  Gain : Gain  Gain=Lks
  Gain1 : Gain  Gain=Rs
  Gain2 : Gain  Gain=np
  Product : Product
  Product1 : Product
  Subsystem : Subsystem
  Te : Outport
  Yrab : Outport  Port=2
  Ysab : Outport  Port=3
  wires:
  Complex to Real-Imag1/2 -> Product1/1  "isb"
  Gain2/1 -> Te/1
  Add2/1 -> Gain2/1
  Product/1 -> Add2/2
  Product1/1 -> Add2/1
  Complex to Real-Imag1/1 -> Product/1  "isa"
  Complex to Real-Imag/2 -> Product/2  "Ysa"
  Complex to Real-Imag/1 -> Product1/2  "Ysa"
  isab/1 -> Gain1/1, Gain/1, Complex to Real-Imag1/1
  Gain/1 -> Add1/2
  Gain1/1 -> Add/2
  vsab/1 -> Add/1
  Add1/1 -> Yrab/1
  Add/1 -> Subsystem/1(In1)
  Subsystem/1(Ysab) -> Ysab/1, Add1/1, Complex to Real-Imag/1  "Ysab"

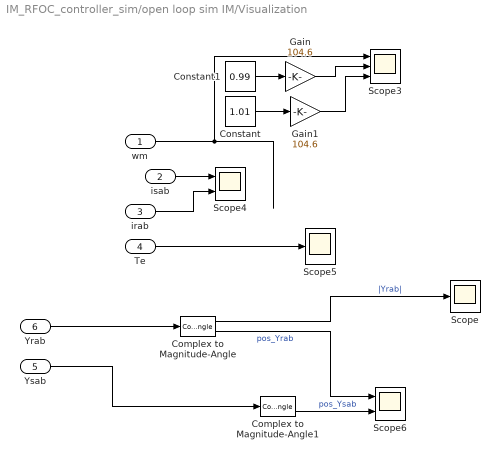
== system IM_RFOC_controller_sim/open loop sim IM/Visualization ==
  wm : Inport
  isab : Inport  Port=2
  irab : Inport  Port=3
  Te : Inport  Port=4
  Ysab : Inport  Port=5
  Yrab : Inport  Port=6
  Complex to Magnitude-Angle : ComplexToMagnitudeAngle
  Complex to Magnitude-Angle1 : ComplexToMagnitudeAngle
  Constant : Constant  Value=1.01
  Constant1 : Constant  Value=0.99
  Gain : Gain  Gain=104.6
  Gain1 : Gain  Gain=104.6
  Scope : Scope
  Scope3 : Scope  NumInputPorts=3
  Scope4 : Scope  NumInputPorts=2
  Scope5 : Scope
  Scope6 : Scope  NumInputPorts=2
  wires:
  Complex to Magnitude-Angle/1 -> Scope/1  "|Yrab|"
  wm/1 -> Scope3/1
  Constant1/1 -> Gain/1
  Gain1/1 -> Scope3/3
  Constant/1 -> Gain1/1
  irab/1 -> Scope4/2
  Complex to Magnitude-Angle/2 -> Scope6/1  "pos_Yrab"
  Gain/1 -> Scope3/2
  Complex to Magnitude-Angle1/2 -> Scope6/2  "pos_Ysab"
  Te/1 -> Scope5/1
  Yrab/1 -> Complex to Magnitude-Angle/1
  isab/1 -> Scope4/1
  Ysab/1 -> Complex to Magnitude-Angle1/1

== system IM_RFOC_controller_sim/open loop sim IM/IM/Subsystem ==
  note: to avoid numerical issues
  In1 : Inport
  Complex to Real-Imag6 : ComplexToRealImag
  Integrator3 : Integrator
  Integrator4 : Integrator
  Real-Imag to Complex : RealImagToComplex
  Ysab : Outport
  wires:
  In1/1 -> Complex to Real-Imag6/1
  Complex to Real-Imag6/2 -> Integrator4/1
  Complex to Real-Imag6/1 -> Integrator3/1
  Integrator3/1 -> Real-Imag to Complex/1
  Real-Imag to Complex/1 -> Ysab/1  "Ysab"
  Integrator4/1 -> Real-Imag to Complex/2

== system IM_RFOC_controller_sim/open loop sim IM/IM/integrator ==
  In1 : Inport
  Complex to Real-Imag7 : ComplexToRealImag
  Integrator1 : Integrator
  Integrator5 : Integrator
  Real-Imag to Complex1 : RealImagToComplex
  Yrab : Outport
  wires:
  Complex to Real-Imag7/2 -> Integrator5/1
  Integrator1/1 -> Real-Imag to Complex1/1
  Real-Imag to Complex1/1 -> Yrab/1  "Yrab"
  Integrator5/1 -> Real-Imag to Complex1/2
  Complex to Real-Imag7/1 -> Integrator1/1
  In1/1 -> Complex to Real-Imag7/1

== system IM_RFOC_controller_sim/open loop sim IM/VI estimator4/Subsystem ==
  note: to avoid numerical issues
  In1 : Inport
  Complex to Real-Imag6 : ComplexToRealImag
  Integrator3 : Integrator
  Integrator4 : Integrator
  Real-Imag to Complex : RealImagToComplex
  Ysab : Outport
  wires:
  Integrator4/1 -> Real-Imag to Complex/2
  Real-Imag to Complex/1 -> Ysab/1  "Ysab"
  Integrator3/1 -> Real-Imag to Complex/1
  Complex to Real-Imag6/1 -> Integrator3/1
  Complex to Real-Imag6/2 -> Integrator4/1
  In1/1 -> Complex to Real-Imag6/1

== matlab function IM_RFOC_controller_sim/Subsystem/MATLAB Function ==
  data: t input; y output
function y = fcn(t)
wm_n = 104.6;
if t<0
    y=0;
elseif t>=0 && t<20
    y = t*0.005*wm_n; 
elseif t>=20 && t<30
    y = 0.1*wm_n;
elseif t>=30 && t<40
    y = t*0.01*wm_n-0.2*wm_n;
else
    y = 0.2*wm_n;
end
